simulink model "teil_diff_2"  (Simulink 6.1)
settings: Solver=ode45  StartTime=0.0  StopTime=10.0  RelTol=1e-3
values from neighbouring files (symbols this model uses):
  delay = verz(Typ)    [analog_hp11.m]    (also in analog_hp12.m; analog_tp11.m; analog_tp12.m; analog_tp2.m = 0.001)
  frausch = 250    [analog_bp3.m]    (also in analog_tp2.m = 500)
  h1 = firpm(128,f,m)    [CFIR_1.m]    (also in G722_1.m = (-1).^(0:L-1).*h0; audio_test1.m = han(:,2); audio_test2.m = han(:,2))
  K = [Krausch, K1, K2, K3, Krechteck, Kdreieck]    [analog_tp2.m]
  Ts = 1/fs    (= 6.25e-05)    [G722_1.m]    (also in adaptiv_2.m = 0.001; adaptiv_3.m = 0.001; adaptiv_4.m = 0.001; adaptiv_5.m = 0.001)
undefined symbols (not defined in the file or in its folder): fst
libraries: dsparch4 x1
settings Model: Creator=svenhoffmann  LastModifiedBy=svenhoffmann  ExtModeAutoUpdateStatusClock=off
settings DebuggingCC: SolverPrmCheckMsg=warning

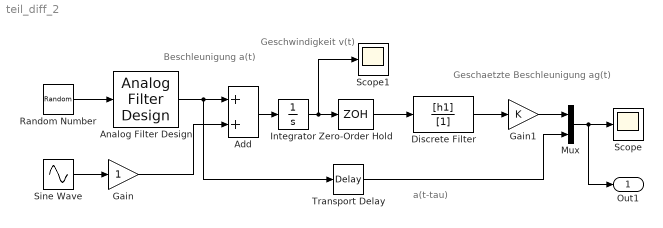
== system teil_diff_2 ==
  note: Beschleunigung
      | a(t)
  note: Geschwindigkeit
      | v(t)
  note: a(t-tau)
  note: Geschaetzte
      | Beschleunigung
      | ag(t)
  Add : Sum  OutScaling=2^-10
  Analog Filter Design : dsparch4/Analog Filter Design  method=Butterworth  filttype=Lowpass  N=8  Wlo=2*pi*frausch  Whi=80  Rp=2  Rs=40
  Discrete Filter : DiscreteFilter  Numerator=[h1]  Denominator=[1]  SampleTime=Ts
  Gain : Gain
  Gain1 : Gain  Gain=K
  Integrator : Integrator
  Mux : Mux  Inputs=2
  Random Number : RandomNumber  SampleTime=0
  Scope : Scope
  Scope1 : Scope
  Sine Wave : Sin  Frequency=2*pi*fst  SampleTime=0
  Transport Delay : TransportDelay  DelayTime=delay
  Zero-Order Hold : ZeroOrderHold  SampleTime=Ts
  Out1 : Outport
  wires:
  Random Number/1 -> Analog Filter Design/1
  Analog Filter Design/1 -> Add/1, Transport Delay/1
  Sine Wave/1 -> Gain/1
  Gain/1 -> Add/2
  Add/1 -> Integrator/1
  Integrator/1 -> Zero-Order Hold/1, Scope1/1
  Zero-Order Hold/1 -> Discrete Filter/1
  Discrete Filter/1 -> Gain1/1
  Gain1/1 -> Mux/1
  Mux/1 -> Scope/1, Out1/1
  Transport Delay/1 -> Mux/2
